simulink model "DQN_ABC_Test"  (R2023b)
settings: Solver=ode23tb  StartTime=0.0  StopTime=0.1  FixedStep=Ts  RelTol=1e-3
values from neighbouring files (symbols this model uses):
  Carm = 3.76    [DQn_ABC_Test_calc.m]
  L = Ld + Lm    [DQn_ABC_Test_calc.m]
  La = 1e-3    (= 0.001)    [DQn_ABC_Test_calc.m]
  Lb = 2*La    (= 0.002)    [DQn_ABC_Test_calc.m]
  Lc = 0.5*La    (= 0.0005)    [DQn_ABC_Test_calc.m]
  N = 1    [DQn_ABC_Test_calc.m]
  R = Rd + Rm    [DQn_ABC_Test_calc.m]
  Ra = 1.64    [DQn_ABC_Test_calc.m]
  Rb = 1.4*Ra    (= 2.296)    [DQn_ABC_Test_calc.m]
  Rc = 2.8*Ra    (= 4.592)    [DQn_ABC_Test_calc.m]
  Ta_dqn = oDP.Ta_dqn    [DQn_ABC_Test_calc.m]
  Ts = 50e-6    (= 5e-05)    [DQn_ABC_Test_calc.m]
  Ts_dqn = Ts    (= 5e-05)    [DQn_ABC_Test_calc.m]
  Ts_emt = Ts    (= 5e-05)    [DQn_ABC_Test_calc.m]
  Ws = 2*pi*f    (= 314.159265359)    [DQn_ABC_Test_calc.m]
undefined symbols (not defined in the file or in its folder): DiscIntNeverNeededParam, i, Xdcpnz, Xdcpnz_c, Xpnz, Ydcpnz, Ydcpnz_c, Ypnz
libraries: DQN_Lib x81, spsCurrentMeasurementLib x9, spsControlledVoltageSourceLib x9, spsSeriesRLCBranchLib x6, spsGroundLib x6, simulink x3, spsMutualInductanceLib x1, spspowerguiLib x1
(part 4 of 6)

== matlab function DQN_ABC_Test/Der_DQNc_Mat ==
  data: Xpnz input; N parameter; Zpnz output; w parameter; EMT parameter; Ts parameter; Init parameter
function Zpnz    = fMultDQNc(Xpnz, N, w, EMT, Ts, Init)
    Zpnz = complex(zeros(3,N+1));

    sX = size(Xpnz,2);
    Xpnz = [Xpnz zeros(3,N+1-sX)];

    persistent Xpnz_old;
    persistent Zpnz_old;
    persistent dt2;


    if(isempty(Xpnz_old)) 
        Xpnz_old = complex(zeros(3,N+1));
        Zpnz_old = complex(zeros(3,N+1));
        dt2 = 0.5*Ts;

    end


    Zpnz(:,1) = dt2*(Xpnz(:,1)+Xpnz_old(:,1)) + Zpnz_old(:,1);

    Xpnz_old(:,1) = Xpnz(:,1);
    Zpnz_old(:,1) = Zpnz(:,1);

    for h = 2 : N + 1
        wn = (h-1)*w;
        if(EMT)
            Zpnz(:,h) = dt2*(Xpnz(:,h)+Xpnz_old(:,h)) + Zpnz_old(:,h);
            Xpnz_old(:,h) = Xpnz(:,h);
            Zpnz_old(:,h) = Zpnz(:,h);
            
        end

        Zpnz(:,h) = Zpnz(:,h) - 1i*Xpnz(:,h)/wn;


    end

    
end

== matlab function DQN_ABC_Test/Int_DQNc_Mat2 ==
  settings: updateMethod=DISCRETE
  data: Xpnz input; N parameter; dt parameter; w parameter; InitInt parameter; Zpnz output; R parameter; iL parameter
function Zpnz    = Int_DQN_Mat(Xpnz, N, dt, w, InitInt, R, iL)

    nrSig = 1;

    Zpnz = complex(zeros(3,N+1));

    persistent Zpnz_old;
    persistent Xpnz_old;
    persistent Krl1;
    persistent Krl2;
    persistent dt2;

        
        
    if(isempty(Zpnz_old)) 
    
        a = -0.5+0.866i;
        a2 = -0.5-0.866i;
        Sas = [1,a,a2;1,a2,a;1,1,1]/3;
        
        Zpnz_old = complex(zeros(3,N+1));
        Xpnz_old = complex(zeros(3,N+1));
        
        if(~isempty(InitInt))
        Zpnz_old(:,1) = Sas * InitInt;
        
        end
        dt2 = dt/2;
        SW = 0;

        R = 1;
        iL = 1;

        if(SW)
            Krl1 = (iL/(1+dt2*R*iL));
            Krl2 = (1-dt2*R*iL)/(1+dt2*R*iL);
        else
            Krl1 = 1;
            Krl2 = 1;
        end
            
    end
       
    
    for k = 1 : nrSig
    
        Zpnz(:,1) = dt2*(Xpnz(:,1)+Xpnz_old(:,1)) + Zpnz_old(:,1);

        Xpnz_old(:,1) = Xpnz(:,1);
        Zpnz_old(:,1) = Zpnz(:,1);


        if(N>0)

            for i = 1 : N
                wn =  i * w; 
                wndt2 = wn*dt2;

                A = 2*dt2/(1+wndt2^2);
                B = (1-wndt2^2)/(1+wndt2^2);

                %%% POS %%%
                Zpnz(1,i+1) =     Krl1*A*(real(Xpnz(1,i+1))+wndt2*imag(Xpnz(1,i+1)))+Krl2*(B*real(Zpnz_old(1,i+1))+A*wn*imag(Zpnz_old(1,i+1))) ...
                            + 1i*(Krl1*A*(imag(Xpnz(1,i+1))-wndt2*real(Xpnz(1,i+1)))+Krl2*(B*imag(Zpnz_old(1,i+1))-A*wn*real(Zpnz_old(1,i+1))));

                %%% NEG %%%
                Zpnz(2,i+1) =     Krl1*A*(real(Xpnz(2,i+1))+wndt2*imag(Xpnz(2,i+1)))+Krl2*(B*real(Zpnz_old(2,i+1))+A*wn*imag(Zpnz_old(2,i+1))) ...
                            + 1i*(Krl1*A*(imag(Xpnz(2,i+1))-wndt2*real(Xpnz(2,i+1)))+Krl2*(B*imag(Zpnz_old(2,i+1))-A*wn*real(Zpnz_old(2,i+1))));

                %%% ZERO %%%
                Zpnz(3,i+1) =     Krl1*A*(real(Xpnz(3,i+1))+wndt2*imag(Xpnz(3,i+1)))+Krl2*(B*real(Zpnz_old(3,i+1))+A*wn*imag(Zpnz_old(3,i+1))) ...
                            + 1i*(Krl1*A*(imag(Xpnz(3,i+1))-wndt2*real(Xpnz(3,i+1)))+Krl2*(B*imag(Zpnz_old(3,i+1))-A*wn*real(Zpnz_old(3,i+1))));


                Zpnz_old(:,i+1) = Zpnz(:,i+1);


            end

        end

    end
end

== matlab function DQN_ABC_Test/Gain_DQNc_Mat2 ==
  data: Xpnz input; Ypnz output; Rabc parameter; chkInv parameter; HRM parameter
function Ypnz  = Gain_Mat2(Xpnz, Rabc, chkInv, HRM)
    persistent Rpnz;
    %persistent nrInp;
    persistent nrOut;

    mrows = size(Rabc,1)/3; %signal size
    mcols = size(Rabc,2)/3; %signal size

    nrInp = size(Rabc,1);

    % Ypnz = complex(zeros(nrInp, HRM+1));


    if(isempty(Rpnz)) 

        Rpnz = complex(zeros(3*mrows,3*mcols));
        a = -0.5+0.866i;
        a2 = -0.5-0.866i;
        Sas = [1,a,a2;1,a2,a;1,1,1]/3;
        %Ssa = eye(3)/(Sas);
        %nrInp = size(Xpnz,1) / 3;

        for i = 1 : mrows
            for j = 1 : mcols
                Rpnz((1:3) + (i-1)*3,(1:3) + (j-1)*3) = Sas*Rabc((1:3) + (i-1)*3,(1:3) + (j-1)*3)/Sas;
            end
        end

        if(chkInv)
            %Rpnz((1:3) + (i-1)*3,(1:3) + (j-1)*3) = eye(3)/Rpnz((1:3) + (i-1)*3,(1:3) + (j-1)*3);
            Rpnz = eye(3*mrows,3*mcols)/Rpnz;
        end

    end




    
    Ypnz = Rpnz*Xpnz;

end

== matlab function DQN_ABC_Test/Int_DQNc_Mat4 ==
  settings: updateMethod=DISCRETE
  data: Xpnz input; N parameter; dt parameter; w parameter; InitInt parameter; Zpnz output; R parameter; iL parameter; swFeed parameter
function Zpnz    = Int_DQN_Mat(Xpnz, N, dt, w, InitInt, R, iL, swFeed)


    nrSig = size(Xpnz,1)/3;
    Zpnz = complex(zeros(nrSig*3,N+1));

    persistent Zpnz_old;
    persistent Xpnz_old;
    persistent Krl1;
    persistent Krl2;
    persistent dt2;
        
    if(isempty(Zpnz_old)) 
    

        Zpnz_old = complex(zeros(nrSig*3,N+1));
        Xpnz_old = complex(zeros(nrSig*3,N+1));
        dt2 = dt/2;

        if(swFeed)
            mrows = size(R,1)/3; %signal size
            mcols = size(R,2)/3; %signal size

            szMatR = size(R,1);
            szMatiL = size(iL,1);

            if(szMatiL ~= szMatR || size(R,1) ~= size(R,2) || size(iL,1) ~= size(iL,2))
                error('[Int_DQN_Mat/swFeedback] check matrix sizes!');
            end
    
            Rpnz = complex(zeros(3*mrows,3*mcols));
            iLpnz = complex(zeros(3*mrows,3*mcols));

            a = -0.5+0.866i;
            a2 = -0.5-0.866i;
            Sas = [1,a,a2;1,a2,a;1,1,1]/3;
    
            for i = 1 : mrows
                for j = 1 : mcols
                     Rpnz((1:3) + (i-1)*3,(1:3) + (j-1)*3) = Sas*R((1:3) + (i-1)*3,(1:3) + (j-1)*3)/Sas;
                    iLpnz((1:3) + (i-1)*3,(1:3) + (j-1)*3) = Sas*iL((1:3) + (i-1)*3,(1:3) + (j-1)*3)/Sas;

                    Rpnz((1:3) + (i-1)*3,(1:3) + (j-1)*3) = diag(diag(real(Rpnz((1:3) + (i-1)*3,(1:3) + (j-1)*3))));
                    iLpnz((1:3) + (i-1)*3,(1:3) + (j-1)*3) = diag(diag(real(iLpnz((1:3) + (i-1)*3,(1:3) + (j-1)*3))));

                end
            end

            Rpnz = real(Rpnz);
            iLpnz = real(iLpnz);

            Krl1 = (iLpnz/(eye(szMatR)+dt2*Rpnz*iLpnz));
            Krl2 = (eye(szMatR)-dt2*Rpnz*iLpnz)/(eye(szMatR)+dt2*Rpnz*iLpnz);

        
            if(~isempty(InitInt))
                % Zpnz_old = x0;
                if(mod(numel(InitInt),3)~=0) error('[SS_DQNc_Mat] x0 vector with wrong size --> needs to be a multiple of 3!'); end
        
                for k = 1 : numel(InitInt)/3
                    Zpnz_old((k-1)*3+1:(k-1)*3+3,1) = Sas*InitInt((k-1)*3+1:(k-1)*3+3);
                end
            end



        else
            Krl1 = 1;
            Krl2 = 1;
        end
            
    end

    if(swFeed)
        Zpnz(:,1) = Krl1*dt2*(Xpnz(:,1)+Xpnz_old(:,1))+Krl2*Zpnz_old(:,1);
    else
        Zpnz(:,1) = dt2*(Xpnz(:,1)+Xpnz_old(:,1))+Zpnz_old(:,1);
    end

    Xpnz_old(:,1) = Xpnz(:,1);
    Zpnz_old(:,1) = Zpnz(:,1);

    for i = 1 : N
        if(N>0)
            wn =  i * w; 
            wndt2 = wn*dt2;

            A = 2*dt2/(1+wndt2^2);
            B = (1-wndt2^2)/(1+wndt2^2);

            if(swFeed)

                Zpnz(:,i+1) =      Krl1*A*(real(Xpnz(:,i+1))+wndt2*imag(Xpnz(:,i+1)))+Krl2*(B*real(Zpnz_old(:,i+1))+A*wn*imag(Zpnz_old(:,i+1))) ...
                             + 1i*(Krl1*A*(imag(Xpnz(:,i+1))-wndt2*real(Xpnz(:,i+1)))+Krl2*(B*imag(Zpnz_old(:,i+1))-A*wn*real(Zpnz_old(:,i+1))));
            else
                Zpnz(:,i+1) =      A*(real(Xpnz(:,i+1))+wndt2*imag(Xpnz(:,i+1)))+(B*real(Zpnz_old(:,i+1))+A*wn*imag(Zpnz_old(:,i+1))) ...
                             + 1i*(A*(imag(Xpnz(:,i+1))-wndt2*real(Xpnz(:,i+1)))+(B*imag(Zpnz_old(:,i+1))-A*wn*real(Zpnz_old(:,i+1))));
            end

            Zpnz_old(:,i+1) = Zpnz(:,i+1);

        end
    end


end
